simulink model "test_circuit_FMI"  (R2022a)
settings: Solver=FixedStepAuto  StartTime=0.0  StopTime=10.0  RelTol=1e-3
libraries: fl_lib x7, nesl_utility x5, spsControlledCurrentSourceLib x1, spsControlledVoltageSourceLib x1, spsCurrentMeasurementLib x1, spsGroundLib x1, spsParallelRLCBranchLib x1, spsSeriesRLCBranchLib x1, spsVoltageMeasurementLib x1, spspowerguiLib x1
(part 1 of 2)
settings Model: Creator=lordx  LastModifiedBy=lordx
settings SolverCC: ZeroCrossControl=EnableAll
settings OptimizationCC: DefaultParameterBehavior=Inlined  EnhancedBackFolding=on  PassReuseOutputArgsAs=Individual arguments  OptimizeBlockOrder=speed  DifferentSizesBufferReuse=on  OptimizationCustomize=off  EfficientTunableParamExpr=on
settings DebuggingCC: ParameterTunabilityLossMsg=error
settings HardwareCC: TargetBitPerPointer=64  TargetBitPerSizeT=64  TargetBitPerPtrDiffT=64  TargetLongLongMode=on  TargetIntDivRoundTo=Zero  TargetEndianess=LittleEndian  TargetWordSize=64  TargetHWDeviceType=MATLAB Host  ProdEqTarget=off
settings ModelReferenceCC: UpdateModelReferenceTargets=Force  EnableRefExpFcnMdlSchedulingChecks=off  ModelReferenceNumInstancesAllowed=Zero  PropagateSignalLabelsOutOfModel=off
settings SFSimCC: SimUserSources="\"F:\\GitHubRepos\\FMI_test_3\\test_circuit_FMI\\sources\\pm_printf.c\" \"F:\\GitHubRepos\\FMI_test_3\\test_circuit_FMI\\sources\\rt_backsubrr_dbl.c\" \"F:\\GitHubRepos\\FMI_test_3\\test_circuit_FMI\\sources\\rt_forwardsubrr_dbl.c\" \"F:\\GitHubRepos\\FMI_test_3\\test_circuit_FMI\\sources\\rt_lu_real.c\" \"F:\\GitHubRepos\\FMI_test_3\\test_circuit_FMI\\sources\\rt_matrixlib_dbl.c\" \"F:\\GitHubRepos\\FMI_test_3\\test_circuit_FMI\\sources\\test_circuit_FMI.c\" \"F:\\GitHubRepos\\FMI_test_3\\test_circuit_FMI\\sources\\test_circuit_FMI_data.c\" \"F:\\GitHubRepos\\FMI_test_3\\test_circuit_FMI\\sources\\RTWCG_FMU_util.c\" \"F:\\GitHubRepos\\FMI_test_3\\test_circuit_FMI\\sources\\test_circuit_FMI_fmu.c\" \"F:\\GitHubRepos\\FMI_test_3\\test_circuit_FMI\\sources\\ssc_sli_0267402d.c\" \"F:\\GitHubRepos\\FMI_test_3\\test_circuit_FMI\\sources\\ssc_sli_0763c151.c\" \"F:\\GitHubRepos\\FMI_test_3\\test_circuit_FMI\\sources\\ssc_sli_0bd269e6.c\" \"F:\\GitHubRepos\\FMI_test_3\\test_circuit_FMI\\sources\\ssc_sli_0d6d0780.c\" \"F:\\GitHubRepos\\FMI_test_3\\test_circuit_FMI\\sources\\ssc_sli_136b443c.c\" \"F:\\GitHubRepos\\FMI_test_3\\test_circuit_FMI\\sources\\ssc_sli_136f97a1.c\" \"F:\\GitHubRepos\\FMI_test_3\\test_circuit_FMI\\sources\\ssc_sli_140b3534.c\" \"F:\\GitHubRepos\\FMI_test_3\\test_circuit_FMI\\sources\\ssc_sli_15d5f6ce.c\" \"F:\\GitHubRepos\\FMI_test_3\\test_circuit_FMI\\sources\\ssc_sli_1c690f90.c\" \"F:\\GitHubRepos\\FMI_test_3\\test_circuit_FMI\\sources\\ssc_sli_1db813e8.c\" \"F:\\GitHubRepos\\FMI_test_3\\test_circuit_FMI\\sources\\ssc_sli_256cd4b6.c\" \"F:\\GitHubRepos\\FMI_test_3\\test_circuit_FMI\\sources\\ssc_sli_2bbd58a4.c\" \"F:\\GitHubRepos\\FMI_test_3\\test_circuit_FMI\\sources\\ssc_sli_2f6ea1cd.c\" \"F:\\GitHubRepos\\FMI_test_3\\test_circuit_FMI\\sources\\ssc_sli_360cfd63.c\" \"F:\\GitHubRepos\\FMI_test_3\\test_circuit_FMI\\sources\\ssc_sli_3fb4607e.c\" \"F:\\GitHubRepos\\FMI_test_3\\test_circuit_FMI\\sources\\ssc_sli_40d56d93.c\" \"F:\\GitHubRepos\\FMI_test_3\\test_circuit_FMI\\sources\\ssc_sli_42b14021.c\" \"F:\\GitHubRepos\\FMI_test_3\\test_circuit_FMI\\sources\\ssc_sli_43618287.c\" \"F:\\GitHubRepos\\FMI_test_3\\test_circuit_FMI\\sources\\ssc_sli_466b08dd.c\" \"F:\\GitHubRepos\\FMI_test_3\\test_circuit_FMI\\sources\\ssc_sli_496799bd.c\" \"F:\\GitHubRepos\\FMI_test_3\\test_circuit_FMI\\sources\\ssc_sli_4e028390.c\" \"F:\\GitHubRepos\\FMI_test_3\\test_circuit_FMI\\sources\\ssc_sli_51dbd3b5.c\" \"F:\\GitHubRepos\\FMI_test_3\\test_circuit_FMI\\sources\\ssc_sli_550a4805.c\" \"F:\\GitHubRepos\\FMI_test_3\\test_circuit_FMI\\sources\\ssc_sli_5a0cb974.c\" \"F:\\GitHubRepos\\FMI_test_3\\test_circuit_FMI\\sources\\ssc_sli_5d63aeeb.c\" \"F:\\GitHubRepos\\FMI_test_3\\test_circuit_FMI\\sources\\ssc_sli_62d81790.c\" \"F:\\GitHubRepos\\FMI_test_3\\test_circuit_FMI\\sources\\ssc_sli_77063d8b.c\" \"F:\\GitHubRepos\\FMI_test_3\\test_circuit_FMI\\sources\\ssc_sli_7a618260.c\" \"F:\\GitHubRepos\\FMI_test_3\\test_circuit_FMI\\sources\\ssc_sli_7f65db03.c\" \"F:\\GitHubRepos\\FMI_test_3\\test_circuit_FMI\\sources\\ssc_sli_880e593a.c\" \"F:\\GitHubRepos\\FMI_test_3\\test_circuit_FMI\\sources\\ssc_sli_89d0f30a.c\" \"F:\\GitHubRepos\\FMI_test_3\\test_circuit_FMI\\sources\\ssc_sli_8a64c4e2.c\" \"F:\\GitHubRepos\\FMI_test_3\\test_circuit_FMI\\sources\\ssc_sli_93019ea6.c\" \"F:\\GitHubRepos\\FMI_test_3\\test_circuit_FMI\\sources\\ssc_sli_9abcdb7f.c\" \"F:\\GitHubRepos\\FMI_test_3\\test_circuit_FMI\\sources\\ssc_sli_9b67747c.c\" \"F:\\GitHubRepos\\FMI_test_3\\test_circuit_FMI\\sources\\ssc_sli_9c030181.c\" \"F:\\GitHubRepos\\FMI_test_3\\test_circuit_FMI\\sources\\ssc_sli_c7dda239.c\" \"F:\\GitHubRepos\\FMI_test_3\\test_circuit_FMI\\sources\\ssc_sli_d064c978.c\" \"F:\\GitHubRepos\\FMI_test_3\\test_circuit_FMI\\sources\\ssc_sli_d80c44d2.c\" \"F:\\GitHubRepos\\FMI_test_3\\test_circuit_FMI\\sources\\ssc_sli_dcd66f69.c\" \"F:\\GitHubRepos\\FMI_test_3\\test_circuit_FMI\\sources\\ssc_sli_e66fe6d5.c\" \"F:\\GitHubRepos\\FMI_test_3\\test_circuit_FMI\\sources\\ssc_sli_e7b327bb.c\" \"F:\\GitHubRepos\\FMI_test_3\\test_circuit_FMI\\sources\\ssc_sli_eb0a5702.c\" \"F:\\GitHubRepos\\FMI_test_3\\test_circuit_FMI\\sources\\ssc_sli_edbee55c.c\" \"F:\\GitHubRepos\\FMI_test_3\\test_circuit_FMI\\sources\\ssc_sli_f6bd9cc8.c\" \"F:\\GitHubRepos\\FMI_test_3\\test_circuit_FMI\\sources\\ssc_sli_f9b5dbc5.c\" \"F:\\GitHubRepos\\FMI_test_3\\test_circuit_FMI\\sources\\ssc_sli_fa0ce53e.c\" \"F:\\GitHubRepos\\FMI_test_3\\test_circuit_FMI\\sources\\ssc_sli_fbdf29da.c\" \"F:\\GitHubRepos\\FMI_test_3\\test_circuit_FMI\\sources\\ssc_core_01dcc633.c\" \"F:\\GitHubRepos\\FMI_test_3\\test_circuit_FMI\\sources\\ssc_core_04da2c69.c\" \"F:\\GitHubRepos\\FMI_test_3\\test_circuit_FMI\\sources\\ssc_core_05058dd9.c\" \"F:\\GitHubRepos\\FMI_test_3\\test_circuit_FMI\\sources\\ssc_core_06ba68a6.c\" \"F:\\GitHubRepos\\FMI_test_3\\test_circuit_FMI\\sources\\ssc_core_09b5fa6e.c\" \"F:\\GitHubRepos\\FMI_test_3\\test_circuit_FMI\\sources\\ssc_core_0bd666aa.c\" \"F:\\GitHubRepos\\FMI_test_3\\test_circuit_FMI\\sources\\ssc_core_0d65be6c.c\" \"F:\\GitHubRepos\\FMI_test_3\\test_circuit_FMI\\sources\\ssc_core_0f019bd9.c\" \"F:\\GitHubRepos\\FMI_test_3\\test_circuit_FMI\\sources\\ssc_core_0f0420a6.c\" \"F:\\GitHubRepos\\FMI_test_3\\test_circuit_FMI\\sources\\ssc_core_18bf4d77.c\" \"F:\\GitHubRepos\\FMI_test_3\\test_circuit_FMI\\sources\\ssc_core_1b0cafd5.c\" \"F:\\GitHubRepos\\FMI_test_3\\test_circuit_FMI\\sources\\ssc_core_1c6b0332.c\" \"F:\\GitHubRepos\\FMI_test_3\\test_circuit_FMI\\sources\\ssc_core_1fd25120.c\" \"F:\\GitHubRepos\\FMI_test_3\\test_circuit_FMI\\sources\\ssc_core_24b4cdee.c\" \"F:\\GitHubRepos\\FMI_test_3\\test_circuit_FMI\\sources\\ssc_core_2568b075.c\" \"F:\\GitHubRepos\\FMI_test_3\\test_circuit_FMI\\sources\\ssc_core_280c0222.c\" \"F:\\GitHubRepos\\FMI_test_3\\test_circuit_FMI\\sources\\ssc_core_2cd54448.c\" \"F:\\GitHubRepos\\FMI_test_3\\test_circuit_FMI\\sources\\ssc_core_3169e4b7.c\" \"F:\\GitHubRepos\\FMI_test_3\\test_circuit_FMI\\sources\\ssc_core_32d8b307.c\" \"F:\\GitHubRepos\\FMI_test_3\\test_circuit_FMI\\sources\\ssc_core_3306c008.c\" \"F:\\GitHubRepos\\FMI_test_3\\test_circuit_FMI\\sources\\ssc_core_360a4baf.c\" \"F:\\GitHubRepos\\FMI_test_3\\test_circuit_FMI\\sources\\ssc_core_37d4ea84.c\" \"F:\\GitHubRepos\\FMI_test_3\\test_circuit_FMI\\sources\\ssc_core_40db642d.c\" \"F:\\GitHubRepos\\FMI_test_3\\test_circuit_FMI\\sources\\ssc_core_40dfdbdc.c\" \"F:\\GitHubRepos\\FMI_test_3\\test_circuit_FMI\\sources\\ssc_core_41017299.c\" \"F:\\GitHubRepos\\FMI_test_3\\test_circuit_FMI\\sources\\ssc_core_4666b45b.c\" \"F:\\GitHubRepos\\FMI_test_3\\test_circuit_FMI\\sources\\ssc_core_48b08af1.c\" \"F:\\GitHubRepos\\FMI_test_3\\test_circuit_FMI\\sources\\ssc_core_48b1386a.c\" \"F:\\GitHubRepos\\FMI_test_3\\test_circuit_FMI\\sources\\ssc_core_4965213d.c\" \"F:\\GitHubRepos\\FMI_test_3\\test_circuit_FMI\\sources\\ssc_core_4ad9135b.c\" \"F:\\GitHubRepos\\FMI_test_3\\test_circuit_FMI\\sources\\ssc_core_4db6bd68.c\" \"F:\\GitHubRepos\\FMI_test_3\\test_circuit_FMI\\sources\\ssc_core_4db86fcc.c\" \"F:\\GitHubRepos\\FMI_test_3\\test_circuit_FMI\\sources\\ssc_core_4e03e39d.c\" \"F:\\GitHubRepos\\FMI_test_3\\test_circuit_FMI\\sources\\ssc_core_4e04eecd.c\" \"F:\\GitHubRepos\\FMI_test_3\\test_circuit_FMI\\sources\\ssc_core_4e06e3bd.c\" \"F:\\GitHubRepos\\FMI_test_3\\test_circuit_FMI\\sources\\ssc_core_54d55ae9.c\" \"F:\\GitHubRepos\\FMI_test_3\\test_circuit_FMI\\sources\\ssc_core_5505224d.c\" \"F:\\GitHubRepos\\FMI_test_3\\test_circuit_FMI\\sources\\ssc_core_550b4c41.c\" \"F:\\GitHubRepos\\FMI_test_3\\test_circuit_FMI\\sources\\ssc_core_56b1a2bf.c\" \"F:\\GitHubRepos\\FMI_test_3\\test_circuit_FMI\\sources\\ssc_core_576cd129.c\" \"F:\\GitHubRepos\\FMI_test_3\\test_circuit_FMI\\sources\\ssc_core_59b034b8.c\" \"F:\\GitHubRepos\\FMI_test_3\\test_circuit_FMI\\sources\\ssc_core_5a046b27.c\" \"F:\\GitHubRepos\\FMI_test_3\\test_circuit_FMI\\sources\\ssc_core_5d6ba758.c\" \"F:\\GitHubRepos\\FMI_test_3\\test_circuit_FMI\\sources\\ssc_core_67d1f118.c\" \"F:\\GitHubRepos\\FMI_test_3\\test_circuit_FMI\\sources\\ssc_core_68da074b.c\" \"F:\\GitHubRepos\\FMI_test_3\\test_circuit_FMI\\sources\\ssc_core_6b663a17.c\" \"F:\\GitHubRepos\\FMI_test_3\\test_circuit_FMI\\sources\\ssc_core_6b6b89d2.c\" \"F:\\GitHubRepos\\FMI_test_3\\test_circuit_FMI\\sources\\ssc_core_6dd833f3.c\" \"F:\\GitHubRepos\\FMI_test_3\\test_circuit_FMI\\sources\\ssc_core_7209d3a5.c\" \"F:\\GitHubRepos\\FMI_test_3\\test_circuit_FMI\\sources\\ssc_core_73d9c2b7.c\" \"F:\\GitHubRepos\\FMI_test_3\\test_circuit_FMI\\sources\\ssc_core_76d825be.c\" \"F:\\GitHubRepos\\FMI_test_3\\test_circuit_FMI\\sources\\ssc_core_770cead7.c\" \"F:\\GitHubRepos\\FMI_test_3\\test_circuit_FMI\\sources\\ssc_core_79dd08ab.c\" \"F:\\GitHubRepos\\FMI_test_3\\test_circuit_FMI\\sources\\ssc_core_7a613edb.c\" \"F:\\GitHubRepos\\FMI_test_3\\test_circuit_FMI\\sources\\ssc_core_83db8762.c\" \"F:\\GitHubRepos\\FMI_test_3\\test_circuit_FMI\\sources\\ssc_core_856738f2.c\" \"F:\\GitHubRepos\\FMI_test_3\\test_circuit_FMI\\sources\\ssc_core_8569edc5.c\" \"F:\\GitHubRepos\\FMI_test_3\\test_circuit_FMI\\sources\\ssc_core_89d7fa79.c\" \"F:\\GitHubRepos\\FMI_test_3\\test_circuit_FMI\\sources\\ssc_core_8a6471dc.c\" \"F:\\GitHubRepos\\FMI_test_3\\test_circuit_FMI\\sources\\ssc_core_8cd9cb37.c\" \"F:\\GitHubRepos\\FMI_test_3\\test_circuit_FMI\\sources\\ssc_core_8d0064b8.c\" \"F:\\GitHubRepos\\FMI_test_3\\test_circuit_FMI\\sources\\ssc_core_96061071.c\" \"F:\\GitHubRepos\\FMI_test_3\\test_circuit_FMI\\sources\\ssc_core_97d767fe.c\" \"F:\\GitHubRepos\\FMI_test_3\\test_circuit_FMI\\sources\\ssc_core_990fe1a4.c\" \"F:\\GitHubRepos\\FMI_test_3\\test_circuit_FMI\\sources\\ssc_core_9b607b15.c\" \"F:\\GitHubRepos\\FMI_test_3\\test_circuit_FMI\\sources\\ssc_core_9b671e57.c\" \"F:\\GitHubRepos\\FMI_test_3\\test_circuit_FMI\\sources\\ssc_core_9c016445.c\" \"F:\\GitHubRepos\\FMI_test_3\\test_circuit_FMI\\sources\\ssc_core_9c01d168.c\" \"F:\\GitHubRepos\\FMI_test_3\\test_circuit_FMI\\sources\\ssc_core_9dd110ad.c\" \"F:\\GitHubRepos\\FMI_test_3\\test_circuit_FMI\\sources\\ssc_core_9fb0e229.c\" \"F:\\GitHubRepos\\FMI_test_3\\test_circuit_FMI\\sources\\ssc_core_9fb25b4f.c\" \"F:\\GitHubRepos\\FMI_test_3\\test_circuit_FMI\\sources\\ssc_core_9fb2e56c.c\" \"F:\\GitHubRepos\\FMI_test_3\\test_circuit_FMI\\sources\\ssc_core_a1d393be.c\" \"F:\\GitHubRepos\\FMI_test_3\\test_circuit_FMI\\sources\\ssc_core_a269ab09.c\" \"F:\\GitHubRepos\\FMI_test_3\\test_circuit_FMI\\sources\\ssc_core_a4d4c45e.c\" \"F:\\GitHubRepos\\FMI_test_3\\test_circuit_FMI\\sources\\ssc_core_a4da1d0a.c\" \"F:\\GitHubRepos\\FMI_test_3\\test_circuit_FMI\\sources\\ssc_core_a6b78ccc.c\" \"F:\\GitHubRepos\\FMI_test_3\\test_circuit_FMI\\sources\\ssc_core_a76299bc.c\" \"F:\\GitHubRepos\\FMI_test_3\\test_circuit_FMI\\sources\\ssc_core_a867d880.c\" \"F:\\GitHubRepos\\FMI_test_3\\test_circuit_FMI\\sources\\ssc_core_a9bbaecc.c\" \"F:\\GitHubRepos\\FMI_test_3\\test_circuit_FMI\\sources\\ssc_core_a9bf1ff2.c\" \"F:\\GitHubRepos\\FMI_test_3\\test_circuit_FMI\\sources\\ssc_core_aa09f23c.c\" \"F:\\GitHubRepos\\FMI_test_3\\test_circuit_FMI\\sources\\ssc_core_abd05c18.c\" \"F:\\GitHubRepos\\FMI_test_3\\test_circuit_FMI\\sources\\ssc_core_abd5e7b4.c\" \"F:\\GitHubRepos\\FMI_test_3\\test_circuit_FMI\\sources\\ssc_core_acb64294.c\" \"F:\\GitHubRepos\\FMI_test_3\\test_circuit_FMI\\sources\\ssc_core_acb6462e.c\" \"F:\\GitHubRepos\\FMI_test_3\\test_circuit_FMI\\sources\\ssc_core_b1038cbb.c\" \"F:\\GitHubRepos\\FMI_test_3\\test_circuit_FMI\\sources\\ssc_core_b10e34f4.c\" \"F:\\GitHubRepos\\FMI_test_3\\test_circuit_FMI\\sources\\ssc_core_b2b3b239.c\" \"F:\\GitHubRepos\\FMI_test_3\\test_circuit_FMI\\sources\\ssc_core_b369cd13.c\" \"F:\\GitHubRepos\\FMI_test_3\\test_circuit_FMI\\sources\\ssc_core_b402b40d.c\" \"F:\\GitHubRepos\\FMI_test_3\\test_circuit_FMI\\sources\\ssc_core_b7b88213.c\" \"F:\\GitHubRepos\\FMI_test_3\\test_circuit_FMI\\sources\\ssc_core_b96ebc21.c\" \"F:\\GitHubRepos\\FMI_test_3\\test_circuit_FMI\\sources\\ssc_core_bad68669.c\" \"F:\\GitHubRepos\\FMI_test_3\\test_circuit_FMI\\sources\\ssc_core_bc648043.c\" \"F:\\GitHubRepos\\FMI_test_3\\test_circuit_FMI\\sources\\ssc_core_bfdb08db.c\" \"F:\\GitHubRepos\\FMI_test_3\\test_circuit_FMI\\sources\\ssc_core_c3003040.c\" \"F:\\GitHubRepos\\FMI_test_3\\test_circuit_FMI\\sources\\ssc_core_c5b050d7.c\" \"F:\\GitHubRepos\\FMI_test_3\\test_circuit_FMI\\sources\\ssc_core_c5b63cb2.c\" \"F:\\GitHubRepos\\FMI_test_3\\test_circuit_FMI\\sources\\ssc_core_c607b660.c\" \"F:\\GitHubRepos\\FMI_test_3\\test_circuit_FMI\\sources\\ssc_core_c8d83e88.c\" \"F:\\GitHubRepos\\FMI_test_3\\test_circuit_FMI\\sources\\ssc_core_cab615c8.c\" \"F:\\GitHubRepos\\FMI_test_3\\test_circuit_FMI\\sources\\ssc_core_cabdc251.c\" \"F:\\GitHubRepos\\FMI_test_3\\test_circuit_FMI\\sources\\ssc_core_cc067f58.c\" \"F:\\GitHubRepos\\FMI_test_3\\test_circuit_FMI\\sources\\ssc_core_cc0bcab0.c\" \"F:\\GitHubRepos\\FMI_test_3\\test_circuit_FMI\\sources\\ssc_core_ce6a84bb.c\" \"F:\\GitHubRepos\\FMI_test_3\\test_circuit_FMI\\sources\\ssc_core_d06d763c.c\" \"F:\\GitHubRepos\\FMI_test_3\\test_circuit_FMI\\sources\\ssc_core_d3d34d7c.c\" \"F:\\GitHubRepos\\FMI_test_3\\test_circuit_FMI\\sources\\ssc_core_d4b9397b.c\" \"F:\\GitHubRepos\\FMI_test_3\\test_circuit_FMI\\sources\\ssc_core_d70a6a09.c\" \"F:\\GitHubRepos\\FMI_test_3\\test_circuit_FMI\\sources\\ssc_core_d807fa59.c\" \"F:\\GitHubRepos\\FMI_test_3\\test_circuit_FMI\\sources\\ssc_core_dcda6edd.c\" \"F:\\GitHubRepos\\FMI_test_3\\test_circuit_FMI\\sources\\ssc_core_deb7fd8d.c\" \"F:\\GitHubRepos\\FMI_test_3\\test_circuit_FMI\\sources\\ssc_core_e0d0866d.c\" \"F:\\GitHubRepos\\FMI_test_3\\test_circuit_FMI\\sources\\ssc_core_e2b61d72.c\" \"F:\\GitHubRepos\\FMI_test_3\\test_circuit_FMI\\sources\\ssc_core_e400c1c2.c\" \"F:\\GitHubRepos\\FMI_test_3\\test_circuit_FMI\\sources\\ssc_core_ead8f455.c\" \"F:\\GitHubRepos\\FMI_test_3\\test_circuit_FMI\\sources\\ssc_core_edb836de.c\" \"F:\\GitHubRepos\\FMI_test_3\\test_circuit_FMI\\sources\\ssc_core_ee000fbe.c\" \"F:\\GitHubRepos\\FMI_test_3\\test_circuit_FMI\\sources\\ssc_core_ee01086d.c\" \"F:\\GitHubRepos\\FMI_test_3\\test_circuit_FMI\\sources\\ssc_core_ee0f0141.c\" \"F:\\GitHubRepos\\FMI_test_3\\test_circuit_FMI\\sources\\ssc_core_f9b6dbed.c\" \"F:\\GitHubRepos\\FMI_test_3\\test_circuit_FMI\\sources\\ssc_core_fa09e9e6.c\" \"F:\\GitHubRepos\\FMI_test_3\\test_circuit_FMI\\sources\\ssc_core_fbd34e62.c\" \"F:\\GitHubRepos\\FMI_test_3\\test_circuit_FMI\\sources\\ssc_core_ff06d9a4.c\" \"F:\\GitHubRepos\\FMI_test_3\\test_circuit_FMI\\sources\\ssc_st_7cd93bb6.c\" \"F:\\GitHubRepos\\FMI_test_3\\test_circuit_FMI\\sources\\ssc_st_da6cd8f8.c\" \"F:\\GitHubRepos\\FMI_test_3\\test_circuit_FMI\\sources\\mc_026e4f4b.c\" \"F:\\GitHubRepos\\FMI_test_3\\test_circuit_FMI\\sources\\mc_03b98f6f.c\" \"F:\\GitHubRepos\\FMI_test_3\\test_circuit_FMI\\sources\\mc_0764157d.c\" \"F:\\GitHubRepos\\FMI_test_3\\test_circuit_FMI\\sources\\mc_0bd30dee.c\" \"F:\\GitHubRepos\\FMI_test_3\\test_circuit_FMI\\sources\\mc_0d6fd085.c\" \"F:\\GitHubRepos\\FMI_test_3\\test_circuit_FMI\\sources\\mc_0ed73c49.c\" \"F:\\GitHubRepos\\FMI_test_3\\test_circuit_FMI\\sources\\mc_0edc34e3.c\" \"F:\\GitHubRepos\\FMI_test_3\\test_circuit_FMI\\sources\\mc_10d4ab75.c\" \"F:\\GitHubRepos\\FMI_test_3\\test_circuit_FMI\\sources\\mc_11086079.c\" \"F:\\GitHubRepos\\FMI_test_3\\test_circuit_FMI\\sources\\mc_110e6c6c.c\" \"F:\\GitHubRepos\\FMI_test_3\\test_circuit_FMI\\sources\\mc_1407e917.c\" \"F:\\GitHubRepos\\FMI_test_3\\test_circuit_FMI\\sources\\mc_140e3c4c.c\" \"F:\\GitHubRepos\\FMI_test_3\\test_circuit_FMI\\sources\\mc_15d12d95.c\" \"F:\\GitHubRepos\\FMI_test_3\\test_circuit_FMI\\sources\\mc_15d828ca.c\" \"F:\\GitHubRepos\\FMI_test_3\\test_circuit_FMI\\sources\\mc_220ba961.c\" \"F:\\GitHubRepos\\FMI_test_3\\test_circuit_FMI\\sources\\mc_2565d6e0.c\" \"F:\\GitHubRepos\\FMI_test_3\\test_circuit_FMI\\sources\\mc_2a642f54.c\" \"F:\\GitHubRepos\\FMI_test_3\\test_circuit_FMI\\sources\\mc_2a6a9b24.c\" \"F:\\GitHubRepos\\FMI_test_3\\test_circuit_FMI\\sources\\mc_2a6b417d.c\" \"F:\\GitHubRepos\\FMI_test_3\\test_circuit_FMI\\sources\\mc_2bbf87e3.c\" \"F:\\GitHubRepos\\FMI_test_3\\test_circuit_FMI\\sources\\mc_2cdc96b4.c\" \"F:\\GitHubRepos\\FMI_test_3\\test_circuit_FMI\\sources\\mc_32d501e3.c\" \"F:\\GitHubRepos\\FMI_test_3\\test_circuit_FMI\\sources\\mc_32dc008a.c\" \"F:\\GitHubRepos\\FMI_test_3\\test_circuit_FMI\\sources\\mc_3b6a945d.c\" \"F:\\GitHubRepos\\FMI_test_3\\test_circuit_FMI\\sources\\mc_3e66abdf.c\" \"F:\\GitHubRepos\\FMI_test_3\\test_circuit_FMI\\sources\\mc_4105189f.c\" \"F:\\GitHubRepos\\FMI_test_3\\test_circuit_FMI\\sources\\mc_47b8cebe.c\" \"F:\\GitHubRepos\\FMI_test_3\\test_circuit_FMI\\sources\\mc_47b91db1.c\" \"F:\\GitHubRepos\\FMI_test_3\\test_circuit_FMI\\sources\\mc_4b0301c6.c\" \"F:\\GitHubRepos\\FMI_test_3\\test_circuit_FMI\\sources\\mc_4c6117e3.c\" \"F:\\GitHubRepos\\FMI_test_3\\test_circuit_FMI\\sources\\mc_51d4094e.c\" \"F:\\GitHubRepos\\FMI_test_3\\test_circuit_FMI\\sources\\mc_52623861.c\" \"F:\\GitHubRepos\\FMI_test_3\\test_circuit_FMI\\sources\\mc_52688a58.c\" \"F:\\GitHubRepos\\FMI_test_3\\test_circuit_FMI\\sources\\mc_53b1fc84.c\" \"F:\\GitHubRepos\\FMI_test_3\\test_circuit_FMI\\sources\\mc_53b6fcf3.c\" \"F:\\GitHubRepos\\FMI_test_3\\test_circuit_FMI\\sources\\mc_550847c3.c\" \"F:\\GitHubRepos\\FMI_test_3\\test_circuit_FMI\\sources\\mc_5766048f.c\" \"F:\\GitHubRepos\\FMI_test_3\\test_circuit_FMI\\sources\\mc_59b6e413.c\" \"F:\\GitHubRepos\\FMI_test_3\\test_circuit_FMI\\sources\\mc_5bd2c9c1.c\" \"F:\\GitHubRepos\\FMI_test_3\\test_circuit_FMI\\sources\\mc_5d65cd86.c\" \"F:\\GitHubRepos\\FMI_test_3\\test_circuit_FMI\\sources\\mc_5edd42ef.c\" \"F:\\GitHubRepos\\FMI_test_3\\test_circuit_FMI\\sources\\mc_630208f8.c\" \"F:\\GitHubRepos\\FMI_test_3\\test_circuit_FMI\\sources\\mc_630dda0e.c\" \"F:\\GitHubRepos\\FMI_test_3\\test_circuit_FMI\\sources\\mc_67da200d.c\" \"F:\\GitHubRepos\\FMI_test_3\\test_circuit_FMI\\sources\\mc_67da4f41.c\" \"F:\\GitHubRepos\\FMI_test_3\\test_circuit_FMI\\sources\\mc_6b6d311a.c\" \"F:\\GitHubRepos\\FMI_test_3\\test_circuit_FMI\\sources\\mc_6e61d16c.c\" \"F:\\GitHubRepos\\FMI_test_3\\test_circuit_FMI\\sources\\mc_6fb1c336.c\" \"F:\\GitHubRepos\\FMI_test_3\\test_circuit_FMI\\sources\\mc_7207b6f4.c\" \"F:\\GitHubRepos\\FMI_test_3\\test_circuit_FMI\\sources\\mc_7809a65c.c\" \"F:\\GitHubRepos\\FMI_test_3\\test_circuit_FMI\\sources\\mc_7a613aec.c\" \"F:\\GitHubRepos\\FMI_test_3\\test_circuit_FMI\\sources\\mc_7bbf41f0.c\" \"F:\\GitHubRepos\\FMI_test_3\\test_circuit_FMI\\sources\\mc_7cd58f0b.c\" \"F:\\GitHubRepos\\FMI_test_3\\test_circuit_FMI\\sources\\mc_7cdbe436.c\" \"F:\\GitHubRepos\\FMI_test_3\\test_circuit_FMI\\sources\\mc_7d0547c8.c\" \"F:\\GitHubRepos\\FMI_test_3\\test_circuit_FMI\\sources\\mc_7d099de7.c\" \"F:\\GitHubRepos\\FMI_test_3\\test_circuit_FMI\\sources\\mc_7eb21b39.c\" \"F:\\GitHubRepos\\FMI_test_3\\test_circuit_FMI\\sources\\mc_81b0ada5.c\" \"F:\\GitHubRepos\\FMI_test_3\\test_circuit_FMI\\sources\\mc_81b5717e.c\" \"F:\\GitHubRepos\\FMI_test_3\\test_circuit_FMI\\sources\\mc_81bc7943.c\" \"F:\\GitHubRepos\\FMI_test_3\\test_circuit_FMI\\sources\\mc_870ec75e.c\" \"F:\\GitHubRepos\\FMI_test_3\\test_circuit_FMI\\sources\\mc_89d597cf.c\" \"F:\\GitHubRepos\\FMI_test_3\\test_circuit_FMI\\sources\\mc_90b6aa0a.c\" \"F:\\GitHubRepos\\FMI_test_3\\test_circuit_FMI\\sources\\mc_95b62b73.c\" \"F:\\GitHubRepos\\FMI_test_3\\test_circuit_FMI\\sources\\mc_9ab7d9b0.c\" \"F:\\GitHubRepos\\FMI_test_3\\test_circuit_FMI\\sources\\mc_9b6376d1.c\" \"F:\\GitHubRepos\\FMI_test_3\\test_circuit_FMI\\sources\\mc_9b6c1529.c\" \"F:\\GitHubRepos\\FMI_test_3\\test_circuit_FMI\\sources\\mc_a2647600.c\" \"F:\\GitHubRepos\\FMI_test_3\\test_circuit_FMI\\sources\\mc_a26bab1a.c\" \"F:\\GitHubRepos\\FMI_test_3\\test_circuit_FMI\\sources\\mc_a3b90582.c\" \"F:\\GitHubRepos\\FMI_test_3\\test_circuit_FMI\\sources\\mc_a6b5ed24.c\" \"F:\\GitHubRepos\\FMI_test_3\\test_circuit_FMI\\sources\\mc_a7684938.c\" \"F:\\GitHubRepos\\FMI_test_3\\test_circuit_FMI\\sources\\mc_a865d1dd.c\" \"F:\\GitHubRepos\\FMI_test_3\\test_circuit_FMI\\sources\\mc_acb3fad7.c\" \"F:\\GitHubRepos\\FMI_test_3\\test_circuit_FMI\\sources\\mc_af0bc203.c\" \"F:\\GitHubRepos\\FMI_test_3\\test_circuit_FMI\\sources\\mc_af0cc4c9.c\" \"F:\\GitHubRepos\\FMI_test_3\\test_circuit_FMI\\sources\\mc_b0de9cbc.c\" \"F:\\GitHubRepos\\FMI_test_3\\test_circuit_FMI\\sources\\mc_b2b86ae3.c\" \"F:\\GitHubRepos\\FMI_test_3\\test_circuit_FMI\\sources\\mc_b362c5eb.c\" \"F:\\GitHubRepos\\FMI_test_3\\test_circuit_FMI\\sources\\mc_b7b03d44.c\" \"F:\\GitHubRepos\\FMI_test_3\\test_circuit_FMI\\sources\\mc_b96a0bad.c\" \"F:\\GitHubRepos\\FMI_test_3\\test_circuit_FMI\\sources\\mc_bb0520ee.c\" \"F:\\GitHubRepos\\FMI_test_3\\test_circuit_FMI\\sources\\mc_bdbb9b78.c\" \"F:\\GitHubRepos\\FMI_test_3\\test_circuit_FMI\\sources\\mc_c2dbf4b2.c\" \"F:\\GitHubRepos\\FMI_test_3\\test_circuit_FMI\\sources\\mc_c8d25d23.c\" \"F:\\GitHubRepos\\FMI_test_3\\test_circuit_FMI\\sources\\mc_cab8a1f9.c\" \"F:\\GitHubRepos\\FMI_test_3\\test_circuit_FMI\\sources\\mc_ce6656ce.c\" \"F:\\GitHubRepos\\FMI_test_3\\test_circuit_FMI\\sources\\mc_d20085b7.c\" \"F:\\GitHubRepos\\FMI_test_3\\test_circuit_FMI\\sources\\mc_d9d38185.c\" \"F:\\GitHubRepos\\FMI_test_3\\test_circuit_FMI\\sources\\mc_dbbb14d2.c\" \"F:\\GitHubRepos\\FMI_test_3\\test_circuit_FMI\\sources\\mc_dcdddfae.c\" \"F:\\GitHubRepos\\FMI_test_3\\test_circuit_FMI\\sources\\mc_debb448f.c\" \"F:\\GitHubRepos\\FMI_test_3\\test_circuit_FMI\\sources\\mc_e7b99cf6.c\" \"F:\\GitHubRepos\\FMI_test_3\\test_circuit_FMI\\sources\\mc_e7bc2f1a.c\" \"F:\\GitHubRepos\\FMI_test_3\\test_circuit_FMI\\sources\\mc_e9661c4a.c\" \"F:\\GitHubRepos\\FMI_test_3\\test_circuit_FMI\\sources\\mc_e969ae87.c\" \"F:\\GitHubRepos\\FMI_test_3\\test_circuit_FMI\\sources\\mc_edbf543c.c\" \"F:\\GitHubRepos\\FMI_test_3\\test_circuit_FMI\\sources\\mc_ee000fbe.c\" \"F:\\GitHubRepos\\FMI_test_3\\test_circuit_FMI\\sources\\mc_efdea3a7.c\" \"F:\\GitHubRepos\\FMI_test_3\\test_circuit_FMI\\sources\\mc_f0012953.c\" \"F:\\GitHubRepos\\FMI_test_3\\test_circuit_FMI\\sources\\mc_f00d2f9b.c\" \"F:\\GitHubRepos\\FMI_test_3\\test_circuit_FMI\\sources\\mc_f3be157c.c\" \"F:\\GitHubRepos\\FMI_test_3\\test_circuit_FMI\\sources\\mc_fbd54145.c\" \"F:\\GitHubRepos\\FMI_test_3\\test_circuit_FMI\\sources\\mc_fcb15a9b.c\" \"F:\\GitHubRepos\\FMI_test_3\\test_circuit_FMI\\sources\\mc_fd619d14.c\" \"F:\\GitHubRepos\\FMI_test_3\\test_circuit_FMI\\sources\\mc_fd6341bb.c\" \"F:\\GitHubRepos\\FMI_test_3\\test_circuit_FMI\\sources\\ex_04d5441d.c\" \"F:\\GitHubRepos\\FMI_test_3\\test_circuit_FMI\\sources\\ex_0d6d0784.c\" \"F:\\GitHubRepos\\FMI_test_3\\test_circuit_FMI\\sources\\ex_136645f8.c\" \"F:\\GitHubRepos\\FMI_test_3\\test_circuit_FMI\\sources\\ex_17bc61ac.c\" \"F:\\GitHubRepos\\FMI_test_3\\test_circuit_FMI\\sources\\ex_18b4440a.c\" \"F:\\GitHubRepos\\FMI_test_3\\test_circuit_FMI\\sources\\ex_1b03ca17.c\" \"F:\\GitHubRepos\\FMI_test_3\\test_circuit_FMI\\sources\\ex_2ebcd5b2.c\" \"F:\\GitHubRepos\\FMI_test_3\\test_circuit_FMI\\sources\\ex_316a81de.c\" \"F:\\GitHubRepos\\FMI_test_3\\test_circuit_FMI\\sources\\ex_36012fa7.c\" \"F:\\GitHubRepos\\FMI_test_3\\test_circuit_FMI\\sources\\ex_40d5be33.c\" \"F:\\GitHubRepos\\FMI_test_3\\test_circuit_FMI\\sources\\ex_47b11894.c\" \"F:\\GitHubRepos\\FMI_test_3\\test_circuit_FMI\\sources\\ex_57660158.c\" \"F:\\GitHubRepos\\FMI_test_3\\test_circuit_FMI\\sources\\ex_690b7cd0.c\" \"F:\\GitHubRepos\\FMI_test_3\\test_circuit_FMI\\sources\\ex_6dd8e72d.c\" \"F:\\GitHubRepos\\FMI_test_3\\test_circuit_FMI\\sources\\ex_770385e6.c\" \"F:\\GitHubRepos\\FMI_test_3\\test_circuit_FMI\\sources\\ex_79d100f1.c\" \"F:\\GitHubRepos\\FMI_test_3\\test_circuit_FMI\\sources\\ex_8a6fc761.c\" \"F:\\GitHubRepos\\FMI_test_3\\test_circuit_FMI\\sources\\ex_98d223a6.c\" \"F:\\GitHubRepos\\FMI_test_3\\test_circuit_FMI\\sources\\ex_aed5de1e.c\" \"F:\\GitHubRepos\\FMI_test_3\\test_circuit_FMI\\sources\\ex_b2b40ad5.c\" \"F:\\GitHubRepos\\FMI_test_3\\test_circuit_FMI\\sources\\ex_bb0efd4b.c\" \"F:\\GitHubRepos\\FMI_test_3\\test_circuit_FMI\\sources\\ex_bfdb009c.c\" \"F:\\GitHubRepos\\FMI_test_3\\test_circuit_FMI\\sources\\ex_c9069dae.c\" \"F:\\GitHubRepos\\FMI_test_3\\test_circuit_FMI\\sources\\ex_d9d686a8.c\" \"F:\\GitHubRepos\\FMI_test_3\\test_circuit_FMI\\sources\\ex_debffef2.c\" \"F:\\GitHubRepos\\FMI_test_3\\test_circuit_FMI\\sources\\ex_e40d74b8.c\" \"F:\\GitHubRepos\\FMI_test_3\\test_circuit_FMI\\sources\\ex_eb0d559b.c\" \"F:\\GitHubRepos\\FMI_test_3\\test_circuit_FMI\\sources\\ex_f6bb4c2d.c\" \"F:\\GitHubRepos\\FMI_test_3\\test_circuit_FMI\\sources\\ex_f866102d.c\" \"F:\\GitHubRepos\\FMI_test_3\\test_circuit_FMI\\sources\\slu_stubbed_definitions.c\" \"F:\\GitHubRepos\\FMI_test_3\\test_circuit_FMI\\sources\\pm_09bc42e2.c\" \"F:\\GitHubRepos\\FMI_test_3\\test_circuit_FMI\\sources\\pm_14098e54.c\" \"F:\\GitHubRepos\\FMI_test_3\\test_circuit_FMI\\sources\\pm_26dc3230.c\" \"F:\\GitHubRepos\\FMI_test_3\\test_circuit_FMI\\sources\\pm_4fd5f5b9.c\" \"F:\\GitHubRepos\\FMI_test_3\\test_circuit_FMI\\sources\\pm_fed8c2c9.c\""  SimUserIncludeDirs="\"D:\\Program Files\\Matlab\\rtw\\c\\FMIKit-Simulink-3.0\" \"D:\\Program Files\\Matlab\\rtw\\c\\FMIKit-Simulink-3.0\\include\" \"F:\\GitHubRepos\\FMI_test_3\\test_circuit_FMI\\sources\""  MATLABDynamicMemAlloc=off
settings RTWCC: SystemTargetFile=ert.tlc  TemplateMakefile=ert_default_tmf  GenerateReport=on  RetainRTWFile=on  CustomInclude="\"D:\\Program Files\\Matlab\\rtw\\c\\FMIKit-Simulink-3.0\" \"D:\\Program Files\\Matlab\\rtw\\c\\FMIKit-Simulink-3.0\\include\" \"F:\\GitHubRepos\\FMI_test_3\\test_circuit_FMI\\sources\""  CustomSource="\"F:\\GitHubRepos\\FMI_test_3\\test_circuit_FMI\\sources\\pm_printf.c\" \"F:\\GitHubRepos\\FMI_test_3\\test_circuit_FMI\\sources\\rt_backsubrr_dbl.c\" \"F:\\GitHubRepos\\FMI_test_3\\test_circuit_FMI\\sources\\rt_forwardsubrr_dbl.c\" \"F:\\GitHubRepos\\FMI_test_3\\test_circuit_FMI\\sources\\rt_lu_real.c\" \"F:\\GitHubRepos\\FMI_test_3\\test_circuit_FMI\\sources\\rt_matrixlib_dbl.c\" \"F:\\GitHubRepos\\FMI_test_3\\test_circuit_FMI\\sources\\test_circuit_FMI.c\" \"F:\\GitHubRepos\\FMI_test_3\\test_circuit_FMI\\sources\\test_circuit_FMI_data.c\" \"F:\\GitHubRepos\\FMI_test_3\\test_circuit_FMI\\sources\\RTWCG_FMU_util.c\" \"F:\\GitHubRepos\\FMI_test_3\\test_circuit_FMI\\sources\\test_circuit_FMI_fmu.c\" \"F:\\GitHubRepos\\FMI_test_3\\test_circuit_FMI\\sources\\ssc_sli_0267402d.c\" \"F:\\GitHubRepos\\FMI_test_3\\test_circuit_FMI\\sources\\ssc_sli_0763c151.c\" \"F:\\GitHubRepos\\FMI_test_3\\test_circuit_FMI\\sources\\ssc_sli_0bd269e6.c\" \"F:\\GitHubRepos\\FMI_test_3\\test_circuit_FMI\\sources\\ssc_sli_0d6d0780.c\" \"F:\\GitHubRepos\\FMI_test_3\\test_circuit_FMI\\sources\\ssc_sli_136b443c.c\" \"F:\\GitHubRepos\\FMI_test_3\\test_circuit_FMI\\sources\\ssc_sli_136f97a1.c\" \"F:\\GitHubRepos\\FMI_test_3\\test_circuit_FMI\\sources\\ssc_sli_140b3534.c\" \"F:\\GitHubRepos\\FMI_test_3\\test_circuit_FMI\\sources\\ssc_sli_15d5f6ce.c\" \"F:\\GitHubRepos\\FMI_test_3\\test_circuit_FMI\\sources\\ssc_sli_1c690f90.c\" \"F:\\GitHubRepos\\FMI_test_3\\test_circuit_FMI\\sources\\ssc_sli_1db813e8.c\" \"F:\\GitHubRepos\\FMI_test_3\\test_circuit_FMI\\sources\\ssc_sli_256cd4b6.c\" \"F:\\GitHubRepos\\FMI_test_3\\test_circuit_FMI\\sources\\ssc_sli_2bbd58a4.c\" \"F:\\GitHubRepos\\FMI_test_3\\test_circuit_FMI\\sources\\ssc_sli_2f6ea1cd.c\" \"F:\\GitHubRepos\\FMI_test_3\\test_circuit_FMI\\sources\\ssc_sli_360cfd63.c\" \"F:\\GitHubRepos\\FMI_test_3\\test_circuit_FMI\\sources\\ssc_sli_3fb4607e.c\" \"F:\\GitHubRepos\\FMI_test_3\\test_circuit_FMI\\sources\\ssc_sli_40d56d93.c\" \"F:\\GitHubRepos\\FMI_test_3\\test_circuit_FMI\\sources\\ssc_sli_42b14021.c\" \"F:\\GitHubRepos\\FMI_test_3\\test_circuit_FMI\\sources\\ssc_sli_43618287.c\" \"F:\\GitHubRepos\\FMI_test_3\\test_circuit_FMI\\sources\\ssc_sli_466b08dd.c\" \"F:\\GitHubRepos\\FMI_test_3\\test_circuit_FMI\\sources\\ssc_sli_496799bd.c\" \"F:\\GitHubRepos\\FMI_test_3\\test_circuit_FMI\\sources\\ssc_sli_4e028390.c\" \"F:\\GitHubRepos\\FMI_test_3\\test_circuit_FMI\\sources\\ssc_sli_51dbd3b5.c\" \"F:\\GitHubRepos\\FMI_test_3\\test_circuit_FMI\\sources\\ssc_sli_550a4805.c\" \"F:\\GitHubRepos\\FMI_test_3\\test_circuit_FMI\\sources\\ssc_sli_5a0cb974.c\" \"F:\\GitHubRepos\\FMI_test_3\\test_circuit_FMI\\sources\\ssc_sli_5d63aeeb.c\" \"F:\\GitHubRepos\\FMI_test_3\\test_circuit_FMI\\sources\\ssc_sli_62d81790.c\" \"F:\\GitHubRepos\\FMI_test_3\\test_circuit_FMI\\sources\\ssc_sli_77063d8b.c\" \"F:\\GitHubRepos\\FMI_test_3\\test_circuit_FMI\\sources\\ssc_sli_7a618260.c\" \"F:\\GitHubRepos\\FMI_test_3\\test_circuit_FMI\\sources\\ssc_sli_7f65db03.c\" \"F:\\GitHubRepos\\FMI_test_3\\test_circuit_FMI\\sources\\ssc_sli_880e593a.c\" \"F:\\GitHubRepos\\FMI_test_3\\test_circuit_FMI\\sources\\ssc_sli_89d0f30a.c\" \"F:\\GitHubRepos\\FMI_test_3\\test_circuit_FMI\\sources\\ssc_sli_8a64c4e2.c\" \"F:\\GitHubRepos\\FMI_test_3\\test_circuit_FMI\\sources\\ssc_sli_93019ea6.c\" \"F:\\GitHubRepos\\FMI_test_3\\test_circuit_FMI\\sources\\ssc_sli_9abcdb7f.c\" \"F:\\GitHubRepos\\FMI_test_3\\test_circuit_FMI\\sources\\ssc_sli_9b67747c.c\" \"F:\\GitHubRepos\\FMI_test_3\\test_circuit_FMI\\sources\\ssc_sli_9c030181.c\" \"F:\\GitHubRepos\\FMI_test_3\\test_circuit_FMI\\sources\\ssc_sli_c7dda239.c\" \"F:\\GitHubRepos\\FMI_test_3\\test_circuit_FMI\\sources\\ssc_sli_d064c978.c\" \"F:\\GitHubRepos\\FMI_test_3\\test_circuit_FMI\\sources\\ssc_sli_d80c44d2.c\" \"F:\\GitHubRepos\\FMI_test_3\\test_circuit_FMI\\sources\\ssc_sli_dcd66f69.c\" \"F:\\GitHubRepos\\FMI_test_3\\test_circuit_FMI\\sources\\ssc_sli_e66fe6d5.c\" \"F:\\GitHubRepos\\FMI_test_3\\test_circuit_FMI\\sources\\ssc_sli_e7b327bb.c\" \"F:\\GitHubRepos\\FMI_test_3\\test_circuit_FMI\\sources\\ssc_sli_eb0a5702.c\" \"F:\\GitHubRepos\\FMI_test_3\\test_circuit_FMI\\sources\\ssc_sli_edbee55c.c\" \"F:\\GitHubRepos\\FMI_test_3\\test_circuit_FMI\\sources\\ssc_sli_f6bd9cc8.c\" \"F:\\GitHubRepos\\FMI_test_3\\test_circuit_FMI\\sources\\ssc_sli_f9b5dbc5.c\" \"F:\\GitHubRepos\\FMI_test_3\\test_circuit_FMI\\sources\\ssc_sli_fa0ce53e.c\" \"F:\\GitHubRepos\\FMI_test_3\\test_circuit_FMI\\sources\\ssc_sli_fbdf29da.c\" \"F:\\GitHubRepos\\FMI_test_3\\test_circuit_FMI\\sources\\ssc_core_01dcc633.c\" \"F:\\GitHubRepos\\FMI_test_3\\test_circuit_FMI\\sources\\ssc_core_04da2c69.c\" \"F:\\GitHubRepos\\FMI_test_3\\test_circuit_FMI\\sources\\ssc_core_05058dd9.c\" \"F:\\GitHubRepos\\FMI_test_3\\test_circuit_FMI\\sources\\ssc_core_06ba68a6.c\" \"F:\\GitHubRepos\\FMI_test_3\\test_circuit_FMI\\sources\\ssc_core_09b5fa6e.c\" \"F:\\GitHubRepos\\FMI_test_3\\test_circuit_FMI\\sources\\ssc_core_0bd666aa.c\" \"F:\\GitHubRepos\\FMI_test_3\\test_circuit_FMI\\sources\\ssc_core_0d65be6c.c\" \"F:\\GitHubRepos\\FMI_test_3\\test_circuit_FMI\\sources\\ssc_core_0f019bd9.c\" \"F:\\GitHubRepos\\FMI_test_3\\test_circuit_FMI\\sources\\ssc_core_0f0420a6.c\" \"F:\\GitHubRepos\\FMI_test_3\\test_circuit_FMI\\sources\\ssc_core_18bf4d77.c\" \"F:\\GitHubRepos\\FMI_test_3\\test_circuit_FMI\\sources\\ssc_core_1b0cafd5.c\" \"F:\\GitHubRepos\\FMI_test_3\\test_circuit_FMI\\sources\\ssc_core_1c6b0332.c\" \"F:\\GitHubRepos\\FMI_test_3\\test_circuit_FMI\\sources\\ssc_core_1fd25120.c\" \"F:\\GitHubRepos\\FMI_test_3\\test_circuit_FMI\\sources\\ssc_core_24b4cdee.c\" \"F:\\GitHubRepos\\FMI_test_3\\test_circuit_FMI\\sources\\ssc_core_2568b075.c\" \"F:\\GitHubRepos\\FMI_test_3\\test_circuit_FMI\\sources\\ssc_core_280c0222.c\" \"F:\\GitHubRepos\\FMI_test_3\\test_circuit_FMI\\sources\\ssc_core_2cd54448.c\" \"F:\\GitHubRepos\\FMI_test_3\\test_circuit_FMI\\sources\\ssc_core_3169e4b7.c\" \"F:\\GitHubRepos\\FMI_test_3\\test_circuit_FMI\\sources\\ssc_core_32d8b307.c\" \"F:\\GitHubRepos\\FMI_test_3\\test_circuit_FMI\\sources\\ssc_core_3306c008.c\" \"F:\\GitHubRepos\\FMI_test_3\\test_circuit_FMI\\sources\\ssc_core_360a4baf.c\" \"F:\\GitHubRepos\\FMI_test_3\\test_circuit_FMI\\sources\\ssc_core_37d4ea84.c\" \"F:\\GitHubRepos\\FMI_test_3\\test_circuit_FMI\\sources\\ssc_core_40db642d.c\" \"F:\\GitHubRepos\\FMI_test_3\\test_circuit_FMI\\sources\\ssc_core_40dfdbdc.c\" \"F:\\GitHubRepos\\FMI_test_3\\test_circuit_FMI\\sources\\ssc_core_41017299.c\" \"F:\\GitHubRepos\\FMI_test_3\\test_circuit_FMI\\sources\\ssc_core_4666b45b.c\" \"F:\\GitHubRepos\\FMI_test_3\\test_circuit_FMI\\sources\\ssc_core_48b08af1.c\" \"F:\\GitHubRepos\\FMI_test_3\\test_circuit_FMI\\sources\\ssc_core_48b1386a.c\" \"F:\\GitHubRepos\\FMI_test_3\\test_circuit_FMI\\sources\\ssc_core_4965213d.c\" \"F:\\GitHubRepos\\FMI_test_3\\test_circuit_FMI\\sources\\ssc_core_4ad9135b.c\" \"F:\\GitHubRepos\\FMI_test_3\\test_circuit_FMI\\sources\\ssc_core_4db6bd68.c\" \"F:\\GitHubRepos\\FMI_test_3\\test_circuit_FMI\\sources\\ssc_core_4db86fcc.c\" \"F:\\GitHubRepos\\FMI_test_3\\test_circuit_FMI\\sources\\ssc_core_4e03e39d.c\" \"F:\\GitHubRepos\\FMI_test_3\\test_circuit_FMI\\sources\\ssc_core_4e04eecd.c\" \"F:\\GitHubRepos\\FMI_test_3\\test_circuit_FMI\\sources\\ssc_core_4e06e3bd.c\" \"F:\\GitHubRepos\\FMI_test_3\\test_circuit_FMI\\sources\\ssc_core_54d55ae9.c\" \"F:\\GitHubRepos\\FMI_test_3\\test_circuit_FMI\\sources\\ssc_core_5505224d.c\" \"F:\\GitHubRepos\\FMI_test_3\\test_circuit_FMI\\sources\\ssc_core_550b4c41.c\" \"F:\\GitHubRepos\\FMI_test_3\\test_circuit_FMI\\sources\\ssc_core_56b1a2bf.c\" \"F:\\GitHubRepos\\FMI_test_3\\test_circuit_FMI\\sources\\ssc_core_576cd129.c\" \"F:\\GitHubRepos\\FMI_test_3\\test_circuit_FMI\\sources\\ssc_core_59b034b8.c\" \"F:\\GitHubRepos\\FMI_test_3\\test_circuit_FMI\\sources\\ssc_core_5a046b27.c\" \"F:\\GitHubRepos\\FMI_test_3\\test_circuit_FMI\\sources\\ssc_core_5d6ba758.c\" \"F:\\GitHubRepos\\FMI_test_3\\test_circuit_FMI\\sources\\ssc_core_67d1f118.c\" \"F:\\GitHubRepos\\FMI_test_3\\test_circuit_FMI\\sources\\ssc_core_68da074b.c\" \"F:\\GitHubRepos\\FMI_test_3\\test_circuit_FMI\\sources\\ssc_core_6b663a17.c\" \"F:\\GitHubRepos\\FMI_test_3\\test_circuit_FMI\\sources\\ssc_core_6b6b89d2.c\" \"F:\\GitHubRepos\\FMI_test_3\\test_circuit_FMI\\sources\\ssc_core_6dd833f3.c\" \"F:\\GitHubRepos\\FMI_test_3\\test_circuit_FMI\\sources\\ssc_core_7209d3a5.c\" \"F:\\GitHubRepos\\FMI_test_3\\test_circuit_FMI\\sources\\ssc_core_73d9c2b7.c\" \"F:\\GitHubRepos\\FMI_test_3\\test_circuit_FMI\\sources\\ssc_core_76d825be.c\" \"F:\\GitHubRepos\\FMI_test_3\\test_circuit_FMI\\sources\\ssc_core_770cead7.c\" \"F:\\GitHubRepos\\FMI_test_3\\test_circuit_FMI\\sources\\ssc_core_79dd08ab.c\" \"F:\\GitHubRepos\\FMI_test_3\\test_circuit_FMI\\sources\\ssc_core_7a613edb.c\" \"F:\\GitHubRepos\\FMI_test_3\\test_circuit_FMI\\sources\\ssc_core_83db8762.c\" \"F:\\GitHubRepos\\FMI_test_3\\test_circuit_FMI\\sources\\ssc_core_856738f2.c\" \"F:\\GitHubRepos\\FMI_test_3\\test_circuit_FMI\\sources\\ssc_core_8569edc5.c\" \"F:\\GitHubRepos\\FMI_test_3\\test_circuit_FMI\\sources\\ssc_core_89d7fa79.c\" \"F:\\GitHubRepos\\FMI_test_3\\test_circuit_FMI\\sources\\ssc_core_8a6471dc.c\" \"F:\\GitHubRepos\\FMI_test_3\\test_circuit_FMI\\sources\\ssc_core_8cd9cb37.c\" \"F:\\GitHubRepos\\FMI_test_3\\test_circuit_FMI\\sources\\ssc_core_8d0064b8.c\" \"F:\\GitHubRepos\\FMI_test_3\\test_circuit_FMI\\sources\\ssc_core_96061071.c\" \"F:\\GitHubRepos\\FMI_test_3\\test_circuit_FMI\\sources\\ssc_core_97d767fe.c\" \"F:\\GitHubRepos\\FMI_test_3\\test_circuit_FMI\\sources\\ssc_core_990fe1a4.c\" \"F:\\GitHubRepos\\FMI_test_3\\test_circuit_FMI\\sources\\ssc_core_9b607b15.c\" \"F:\\GitHubRepos\\FMI_test_3\\test_circuit_FMI\\sources\\ssc_core_9b671e57.c\" \"F:\\GitHubRepos\\FMI_test_3\\test_circuit_FMI\\sources\\ssc_core_9c016445.c\" \"F:\\GitHubRepos\\FMI_test_3\\test_circuit_FMI\\sources\\ssc_core_9c01d168.c\" \"F:\\GitHubRepos\\FMI_test_3\\test_circuit_FMI\\sources\\ssc_core_9dd110ad.c\" \"F:\\GitHubRepos\\FMI_test_3\\test_circuit_FMI\\sources\\ssc_core_9fb0e229.c\" \"F:\\GitHubRepos\\FMI_test_3\\test_circuit_FMI\\sources\\ssc_core_9fb25b4f.c\" \"F:\\GitHubRepos\\FMI_test_3\\test_circuit_FMI\\sources\\ssc_core_9fb2e56c.c\" \"F:\\GitHubRepos\\FMI_test_3\\test_circuit_FMI\\sources\\ssc_core_a1d393be.c\" \"F:\\GitHubRepos\\FMI_test_3\\test_circuit_FMI\\sources\\ssc_core_a269ab09.c\" \"F:\\GitHubRepos\\FMI_test_3\\test_circuit_FMI\\sources\\ssc_core_a4d4c45e.c\" \"F:\\GitHubRepos\\FMI_test_3\\test_circuit_FMI\\sources\\ssc_core_a4da1d0a.c\" \"F:\\GitHubRepos\\FMI_test_3\\test_circuit_FMI\\sources\\ssc_core_a6b78ccc.c\" \"F:\\GitHubRepos\\FMI_test_3\\test_circuit_FMI\\sources\\ssc_core_a76299bc.c\" \"F:\\GitHubRepos\\FMI_test_3\\test_circuit_FMI\\sources\\ssc_core_a867d880.c\" \"F:\\GitHubRepos\\FMI_test_3\\test_circuit_FMI\\sources\\ssc_core_a9bbaecc.c\" \"F:\\GitHubRepos\\FMI_test_3\\test_circuit_FMI\\sources\\ssc_core_a9bf1ff2.c\" \"F:\\GitHubRepos\\FMI_test_3\\test_circuit_FMI\\sources\\ssc_core_aa09f23c.c\" \"F:\\GitHubRepos\\FMI_test_3\\test_circuit_FMI\\sources\\ssc_core_abd05c18.c\" \"F:\\GitHubRepos\\FMI_test_3\\test_circuit_FMI\\sources\\ssc_core_abd5e7b4.c\" \"F:\\GitHubRepos\\FMI_test_3\\test_circuit_FMI\\sources\\ssc_core_acb64294.c\" \"F:\\GitHubRepos\\FMI_test_3\\test_circuit_FMI\\sources\\ssc_core_acb6462e.c\" \"F:\\GitHubRepos\\FMI_test_3\\test_circuit_FMI\\sources\\ssc_core_b1038cbb.c\" \"F:\\GitHubRepos\\FMI_test_3\\test_circuit_FMI\\sources\\ssc_core_b10e34f4.c\" \"F:\\GitHubRepos\\FMI_test_3\\test_circuit_FMI\\sources\\ssc_core_b2b3b239.c\" \"F:\\GitHubRepos\\FMI_test_3\\test_circuit_FMI\\sources\\ssc_core_b369cd13.c\" \"F:\\GitHubRepos\\FMI_test_3\\test_circuit_FMI\\sources\\ssc_core_b402b40d.c\" \"F:\\GitHubRepos\\FMI_test_3\\test_circuit_FMI\\sources\\ssc_core_b7b88213.c\" \"F:\\GitHubRepos\\FMI_test_3\\test_circuit_FMI\\sources\\ssc_core_b96ebc21.c\" \"F:\\GitHubRepos\\FMI_test_3\\test_circuit_FMI\\sources\\ssc_core_bad68669.c\" \"F:\\GitHubRepos\\FMI_test_3\\test_circuit_FMI\\sources\\ssc_core_bc648043.c\" \"F:\\GitHubRepos\\FMI_test_3\\test_circuit_FMI\\sources\\ssc_core_bfdb08db.c\" \"F:\\GitHubRepos\\FMI_test_3\\test_circuit_FMI\\sources\\ssc_core_c3003040.c\" \"F:\\GitHubRepos\\FMI_test_3\\test_circuit_FMI\\sources\\ssc_core_c5b050d7.c\" \"F:\\GitHubRepos\\FMI_test_3\\test_circuit_FMI\\sources\\ssc_core_c5b63cb2.c\" \"F:\\GitHubRepos\\FMI_test_3\\test_circuit_FMI\\sources\\ssc_core_c607b660.c\" \"F:\\GitHubRepos\\FMI_test_3\\test_circuit_FMI\\sources\\ssc_core_c8d83e88.c\" \"F:\\GitHubRepos\\FMI_test_3\\test_circuit_FMI\\sources\\ssc_core_cab615c8.c\" \"F:\\GitHubRepos\\FMI_test_3\\test_circuit_FMI\\sources\\ssc_core_cabdc251.c\" \"F:\\GitHubRepos\\FMI_test_3\\test_circuit_FMI\\sources\\ssc_core_cc067f58.c\" \"F:\\GitHubRepos\\FMI_test_3\\test_circuit_FMI\\sources\\ssc_core_cc0bcab0.c\" \"F:\\GitHubRepos\\FMI_test_3\\test_circuit_FMI\\sources\\ssc_core_ce6a84bb.c\" \"F:\\GitHubRepos\\FMI_test_3\\test_circuit_FMI\\sources\\ssc_core_d06d763c.c\" \"F:\\GitHubRepos\\FMI_test_3\\test_circuit_FMI\\sources\\ssc_core_d3d34d7c.c\" \"F:\\GitHubRepos\\FMI_test_3\\test_circuit_FMI\\sources\\ssc_core_d4b9397b.c\" \"F:\\GitHubRepos\\FMI_test_3\\test_circuit_FMI\\sources\\ssc_core_d70a6a09.c\" \"F:\\GitHubRepos\\FMI_test_3\\test_circuit_FMI\\sources\\ssc_core_d807fa59.c\" \"F:\\GitHubRepos\\FMI_test_3\\test_circuit_FMI\\sources\\ssc_core_dcda6edd.c\" \"F:\\GitHubRepos\\FMI_test_3\\test_circuit_FMI\\sources\\ssc_core_deb7fd8d.c\" \"F:\\GitHubRepos\\FMI_test_3\\test_circuit_FMI\\sources\\ssc_core_e0d0866d.c\" \"F:\\GitHubRepos\\FMI_test_3\\test_circuit_FMI\\sources\\ssc_core_e2b61d72.c\" \"F:\\GitHubRepos\\FMI_test_3\\test_circuit_FMI\\sources\\ssc_core_e400c1c2.c\" \"F:\\GitHubRepos\\FMI_test_3\\test_circuit_FMI\\sources\\ssc_core_ead8f455.c\" \"F:\\GitHubRepos\\FMI_test_3\\test_circuit_FMI\\sources\\ssc_core_edb836de.c\" \"F:\\GitHubRepos\\FMI_test_3\\test_circuit_FMI\\sources\\ssc_core_ee000fbe.c\" \"F:\\GitHubRepos\\FMI_test_3\\test_circuit_FMI\\sources\\ssc_core_ee01086d.c\" \"F:\\GitHubRepos\\FMI_test_3\\test_circuit_FMI\\sources\\ssc_core_ee0f0141.c\" \"F:\\GitHubRepos\\FMI_test_3\\test_circuit_FMI\\sources\\ssc_core_f9b6dbed.c\" \"F:\\GitHubRepos\\FMI_test_3\\test_circuit_FMI\\sources\\ssc_core_fa09e9e6.c\" \"F:\\GitHubRepos\\FMI_test_3\\test_circuit_FMI\\sources\\ssc_core_fbd34e62.c\" \"F:\\GitHubRepos\\FMI_test_3\\test_circuit_FMI\\sources\\ssc_core_ff06d9a4.c\" \"F:\\GitHubRepos\\FMI_test_3\\test_circuit_FMI\\sources\\ssc_st_7cd93bb6.c\" \"F:\\GitHubRepos\\FMI_test_3\\test_circuit_FMI\\sources\\ssc_st_da6cd8f8.c\" \"F:\\GitHubRepos\\FMI_test_3\\test_circuit_FMI\\sources\\mc_026e4f4b.c\" \"F:\\GitHubRepos\\FMI_test_3\\test_circuit_FMI\\sources\\mc_03b98f6f.c\" \"F:\\GitHubRepos\\FMI_test_3\\test_circuit_FMI\\sources\\mc_0764157d.c\" \"F:\\GitHubRepos\\FMI_test_3\\test_circuit_FMI\\sources\\mc_0bd30dee.c\" \"F:\\GitHubRepos\\FMI_test_3\\test_circuit_FMI\\sources\\mc_0d6fd085.c\" \"F:\\GitHubRepos\\FMI_test_3\\test_circuit_FMI\\sources\\mc_0ed73c49.c\" \"F:\\GitHubRepos\\FMI_test_3\\test_circuit_FMI\\sources\\mc_0edc34e3.c\" \"F:\\GitHubRepos\\FMI_test_3\\test_circuit_FMI\\sources\\mc_10d4ab75.c\" \"F:\\GitHubRepos\\FMI_test_3\\test_circuit_FMI\\sources\\mc_11086079.c\" \"F:\\GitHubRepos\\FMI_test_3\\test_circuit_FMI\\sources\\mc_110e6c6c.c\" \"F:\\GitHubRepos\\FMI_test_3\\test_circuit_FMI\\sources\\mc_1407e917.c\" \"F:\\GitHubRepos\\FMI_test_3\\test_circuit_FMI\\sources\\mc_140e3c4c.c\" \"F:\\GitHubRepos\\FMI_test_3\\test_circuit_FMI\\sources\\mc_15d12d95.c\" \"F:\\GitHubRepos\\FMI_test_3\\test_circuit_FMI\\sources\\mc_15d828ca.c\" \"F:\\GitHubRepos\\FMI_test_3\\test_circuit_FMI\\sources\\mc_220ba961.c\" \"F:\\GitHubRepos\\FMI_test_3\\test_circuit_FMI\\sources\\mc_2565d6e0.c\" \"F:\\GitHubRepos\\FMI_test_3\\test_circuit_FMI\\sources\\mc_2a642f54.c\" \"F:\\GitHubRepos\\FMI_test_3\\test_circuit_FMI\\sources\\mc_2a6a9b24.c\" \"F:\\GitHubRepos\\FMI_test_3\\test_circuit_FMI\\sources\\mc_2a6b417d.c\" \"F:\\GitHubRepos\\FMI_test_3\\test_circuit_FMI\\sources\\mc_2bbf87e3.c\" \"F:\\GitHubRepos\\FMI_test_3\\test_circuit_FMI\\sources\\mc_2cdc96b4.c\" \"F:\\GitHubRepos\\FMI_test_3\\test_circuit_FMI\\sources\\mc_32d501e3.c\" \"F:\\GitHubRepos\\FMI_test_3\\test_circuit_FMI\\sources\\mc_32dc008a.c\" \"F:\\GitHubRepos\\FMI_test_3\\test_circuit_FMI\\sources\\mc_3b6a945d.c\" \"F:\\GitHubRepos\\FMI_test_3\\test_circuit_FMI\\sources\\mc_3e66abdf.c\" \"F:\\GitHubRepos\\FMI_test_3\\test_circuit_FMI\\sources\\mc_4105189f.c\" \"F:\\GitHubRepos\\FMI_test_3\\test_circuit_FMI\\sources\\mc_47b8cebe.c\" \"F:\\GitHubRepos\\FMI_test_3\\test_circuit_FMI\\sources\\mc_47b91db1.c\" \"F:\\GitHubRepos\\FMI_test_3\\test_circuit_FMI\\sources\\mc_4b0301c6.c\" \"F:\\GitHubRepos\\FMI_test_3\\test_circuit_FMI\\sources\\mc_4c6117e3.c\" \"F:\\GitHubRepos\\FMI_test_3\\test_circuit_FMI\\sources\\mc_51d4094e.c\" \"F:\\GitHubRepos\\FMI_test_3\\test_circuit_FMI\\sources\\mc_52623861.c\" \"F:\\GitHubRepos\\FMI_test_3\\test_circuit_FMI\\sources\\mc_52688a58.c\" \"F:\\GitHubRepos\\FMI_test_3\\test_circuit_FMI\\sources\\mc_53b1fc84.c\" \"F:\\GitHubRepos\\FMI_test_3\\test_circuit_FMI\\sources\\mc_53b6fcf3.c\" \"F:\\GitHubRepos\\FMI_test_3\\test_circuit_FMI\\sources\\mc_550847c3.c\" \"F:\\GitHubRepos\\FMI_test_3\\test_circuit_FMI\\sources\\mc_5766048f.c\" \"F:\\GitHubRepos\\FMI_test_3\\test_circuit_FMI\\sources\\mc_59b6e413.c\" \"F:\\GitHubRepos\\FMI_test_3\\test_circuit_FMI\\sources\\mc_5bd2c9c1.c\" \"F:\\GitHubRepos\\FMI_test_3\\test_circuit_FMI\\sources\\mc_5d65cd86.c\" \"F:\\GitHubRepos\\FMI_test_3\\test_circuit_FMI\\sources\\mc_5edd42ef.c\" \"F:\\GitHubRepos\\FMI_test_3\\test_circuit_FMI\\sources\\mc_630208f8.c\" \"F:\\GitHubRepos\\FMI_test_3\\test_circuit_FMI\\sources\\mc_630dda0e.c\" \"F:\\GitHubRepos\\FMI_test_3\\test_circuit_FMI\\sources\\mc_67da200d.c\" \"F:\\GitHubRepos\\FMI_test_3\\test_circuit_FMI\\sources\\mc_67da4f41.c\" \"F:\\GitHubRepos\\FMI_test_3\\test_circuit_FMI\\sources\\mc_6b6d311a.c\" \"F:\\GitHubRepos\\FMI_test_3\\test_circuit_FMI\\sources\\mc_6e61d16c.c\" \"F:\\GitHubRepos\\FMI_test_3\\test_circuit_FMI\\sources\\mc_6fb1c336.c\" \"F:\\GitHubRepos\\FMI_test_3\\test_circuit_FMI\\sources\\mc_7207b6f4.c\" \"F:\\GitHubRepos\\FMI_test_3\\test_circuit_FMI\\sources\\mc_7809a65c.c\" \"F:\\GitHubRepos\\FMI_test_3\\test_circuit_FMI\\sources\\mc_7a613aec.c\" \"F:\\GitHubRepos\\FMI_test_3\\test_circuit_FMI\\sources\\mc_7bbf41f0.c\" \"F:\\GitHubRepos\\FMI_test_3\\test_circuit_FMI\\sources\\mc_7cd58f0b.c\" \"F:\\GitHubRepos\\FMI_test_3\\test_circuit_FMI\\sources\\mc_7cdbe436.c\" \"F:\\GitHubRepos\\FMI_test_3\\test_circuit_FMI\\sources\\mc_7d0547c8.c\" \"F:\\GitHubRepos\\FMI_test_3\\test_circuit_FMI\\sources\\mc_7d099de7.c\" \"F:\\GitHubRepos\\FMI_test_3\\test_circuit_FMI\\sources\\mc_7eb21b39.c\" \"F:\\GitHubRepos\\FMI_test_3\\test_circuit_FMI\\sources\\mc_81b0ada5.c\" \"F:\\GitHubRepos\\FMI_test_3\\test_circuit_FMI\\sources\\mc_81b5717e.c\" \"F:\\GitHubRepos\\FMI_test_3\\test_circuit_FMI\\sources\\mc_81bc7943.c\" \"F:\\GitHubRepos\\FMI_test_3\\test_circuit_FMI\\sources\\mc_870ec75e.c\" \"F:\\GitHubRepos\\FMI_test_3\\test_circuit_FMI\\sources\\mc_89d597cf.c\" \"F:\\GitHubRepos\\FMI_test_3\\test_circuit_FMI\\sources\\mc_90b6aa0a.c\" \"F:\\GitHubRepos\\FMI_test_3\\test_circuit_FMI\\sources\\mc_95b62b73.c\" \"F:\\GitHubRepos\\FMI_test_3\\test_circuit_FMI\\sources\\mc_9ab7d9b0.c\" \"F:\\GitHubRepos\\FMI_test_3\\test_circuit_FMI\\sources\\mc_9b6376d1.c\" \"F:\\GitHubRepos\\FMI_test_3\\test_circuit_FMI\\sources\\mc_9b6c1529.c\" \"F:\\GitHubRepos\\FMI_test_3\\test_circuit_FMI\\sources\\mc_a2647600.c\" \"F:\\GitHubRepos\\FMI_test_3\\test_circuit_FMI\\sources\\mc_a26bab1a.c\" \"F:\\GitHubRepos\\FMI_test_3\\test_circuit_FMI\\sources\\mc_a3b90582.c\" \"F:\\GitHubRepos\\FMI_test_3\\test_circuit_FMI\\sources\\mc_a6b5ed24.c\" \"F:\\GitHubRepos\\FMI_test_3\\test_circuit_FMI\\sources\\mc_a7684938.c\" \"F:\\GitHubRepos\\FMI_test_3\\test_circuit_FMI\\sources\\mc_a865d1dd.c\" \"F:\\GitHubRepos\\FMI_test_3\\test_circuit_FMI\\sources\\mc_acb3fad7.c\" \"F:\\GitHubRepos\\FMI_test_3\\test_circuit_FMI\\sources\\mc_af0bc203.c\" \"F:\\GitHubRepos\\FMI_test_3\\test_circuit_FMI\\sources\\mc_af0cc4c9.c\" \"F:\\GitHubRepos\\FMI_test_3\\test_circuit_FMI\\sources\\mc_b0de9cbc.c\" \"F:\\GitHubRepos\\FMI_test_3\\test_circuit_FMI\\sources\\mc_b2b86ae3.c\" \"F:\\GitHubRepos\\FMI_test_3\\test_circuit_FMI\\sources\\mc_b362c5eb.c\" \"F:\\GitHubRepos\\FMI_test_3\\test_circuit_FMI\\sources\\mc_b7b03d44.c\" \"F:\\GitHubRepos\\FMI_test_3\\test_circuit_FMI\\sources\\mc_b96a0bad.c\" \"F:\\GitHubRepos\\FMI_test_3\\test_circuit_FMI\\sources\\mc_bb0520ee.c\" \"F:\\GitHubRepos\\FMI_test_3\\test_circuit_FMI\\sources\\mc_bdbb9b78.c\" \"F:\\GitHubRepos\\FMI_test_3\\test_circuit_FMI\\sources\\mc_c2dbf4b2.c\" \"F:\\GitHubRepos\\FMI_test_3\\test_circuit_FMI\\sources\\mc_c8d25d23.c\" \"F:\\GitHubRepos\\FMI_test_3\\test_circuit_FMI\\sources\\mc_cab8a1f9.c\" \"F:\\GitHubRepos\\FMI_test_3\\test_circuit_FMI\\sources\\mc_ce6656ce.c\" \"F:\\GitHubRepos\\FMI_test_3\\test_circuit_FMI\\sources\\mc_d20085b7.c\" \"F:\\GitHubRepos\\FMI_test_3\\test_circuit_FMI\\sources\\mc_d9d38185.c\" \"F:\\GitHubRepos\\FMI_test_3\\test_circuit_FMI\\sources\\mc_dbbb14d2.c\" \"F:\\GitHubRepos\\FMI_test_3\\test_circuit_FMI\\sources\\mc_dcdddfae.c\" \"F:\\GitHubRepos\\FMI_test_3\\test_circuit_FMI\\sources\\mc_debb448f.c\" \"F:\\GitHubRepos\\FMI_test_3\\test_circuit_FMI\\sources\\mc_e7b99cf6.c\" \"F:\\GitHubRepos\\FMI_test_3\\test_circuit_FMI\\sources\\mc_e7bc2f1a.c\" \"F:\\GitHubRepos\\FMI_test_3\\test_circuit_FMI\\sources\\mc_e9661c4a.c\" \"F:\\GitHubRepos\\FMI_test_3\\test_circuit_FMI\\sources\\mc_e969ae87.c\" \"F:\\GitHubRepos\\FMI_test_3\\test_circuit_FMI\\sources\\mc_edbf543c.c\" \"F:\\GitHubRepos\\FMI_test_3\\test_circuit_FMI\\sources\\mc_ee000fbe.c\" \"F:\\GitHubRepos\\FMI_test_3\\test_circuit_FMI\\sources\\mc_efdea3a7.c\" \"F:\\GitHubRepos\\FMI_test_3\\test_circuit_FMI\\sources\\mc_f0012953.c\" \"F:\\GitHubRepos\\FMI_test_3\\test_circuit_FMI\\sources\\mc_f00d2f9b.c\" \"F:\\GitHubRepos\\FMI_test_3\\test_circuit_FMI\\sources\\mc_f3be157c.c\" \"F:\\GitHubRepos\\FMI_test_3\\test_circuit_FMI\\sources\\mc_fbd54145.c\" \"F:\\GitHubRepos\\FMI_test_3\\test_circuit_FMI\\sources\\mc_fcb15a9b.c\" \"F:\\GitHubRepos\\FMI_test_3\\test_circuit_FMI\\sources\\mc_fd619d14.c\" \"F:\\GitHubRepos\\FMI_test_3\\test_circuit_FMI\\sources\\mc_fd6341bb.c\" \"F:\\GitHubRepos\\FMI_test_3\\test_circuit_FMI\\sources\\ex_04d5441d.c\" \"F:\\GitHubRepos\\FMI_test_3\\test_circuit_FMI\\sources\\ex_0d6d0784.c\" \"F:\\GitHubRepos\\FMI_test_3\\test_circuit_FMI\\sources\\ex_136645f8.c\" \"F:\\GitHubRepos\\FMI_test_3\\test_circuit_FMI\\sources\\ex_17bc61ac.c\" \"F:\\GitHubRepos\\FMI_test_3\\test_circuit_FMI\\sources\\ex_18b4440a.c\" \"F:\\GitHubRepos\\FMI_test_3\\test_circuit_FMI\\sources\\ex_1b03ca17.c\" \"F:\\GitHubRepos\\FMI_test_3\\test_circuit_FMI\\sources\\ex_2ebcd5b2.c\" \"F:\\GitHubRepos\\FMI_test_3\\test_circuit_FMI\\sources\\ex_316a81de.c\" \"F:\\GitHubRepos\\FMI_test_3\\test_circuit_FMI\\sources\\ex_36012fa7.c\" \"F:\\GitHubRepos\\FMI_test_3\\test_circuit_FMI\\sources\\ex_40d5be33.c\" \"F:\\GitHubRepos\\FMI_test_3\\test_circuit_FMI\\sources\\ex_47b11894.c\" \"F:\\GitHubRepos\\FMI_test_3\\test_circuit_FMI\\sources\\ex_57660158.c\" \"F:\\GitHubRepos\\FMI_test_3\\test_circuit_FMI\\sources\\ex_690b7cd0.c\" \"F:\\GitHubRepos\\FMI_test_3\\test_circuit_FMI\\sources\\ex_6dd8e72d.c\" \"F:\\GitHubRepos\\FMI_test_3\\test_circuit_FMI\\sources\\ex_770385e6.c\" \"F:\\GitHubRepos\\FMI_test_3\\test_circuit_FMI\\sources\\ex_79d100f1.c\" \"F:\\GitHubRepos\\FMI_test_3\\test_circuit_FMI\\sources\\ex_8a6fc761.c\" \"F:\\GitHubRepos\\FMI_test_3\\test_circuit_FMI\\sources\\ex_98d223a6.c\" \"F:\\GitHubRepos\\FMI_test_3\\test_circuit_FMI\\sources\\ex_aed5de1e.c\" \"F:\\GitHubRepos\\FMI_test_3\\test_circuit_FMI\\sources\\ex_b2b40ad5.c\" \"F:\\GitHubRepos\\FMI_test_3\\test_circuit_FMI\\sources\\ex_bb0efd4b.c\" \"F:\\GitHubRepos\\FMI_test_3\\test_circuit_FMI\\sources\\ex_bfdb009c.c\" \"F:\\GitHubRepos\\FMI_test_3\\test_circuit_FMI\\sources\\ex_c9069dae.c\" \"F:\\GitHubRepos\\FMI_test_3\\test_circuit_FMI\\sources\\ex_d9d686a8.c\" \"F:\\GitHubRepos\\FMI_test_3\\test_circuit_FMI\\sources\\ex_debffef2.c\" \"F:\\GitHubRepos\\FMI_test_3\\test_circuit_FMI\\sources\\ex_e40d74b8.c\" \"F:\\GitHubRepos\\FMI_test_3\\test_circuit_FMI\\sources\\ex_eb0d559b.c\" \"F:\\GitHubRepos\\FMI_test_3\\test_circuit_FMI\\sources\\ex_f6bb4c2d.c\" \"F:\\GitHubRepos\\FMI_test_3\\test_circuit_FMI\\sources\\ex_f866102d.c\" \"F:\\GitHubRepos\\FMI_test_3\\test_circuit_FMI\\sources\\slu_stubbed_definitions.c\" \"F:\\GitHubRepos\\FMI_test_3\\test_circuit_FMI\\sources\\pm_09bc42e2.c\" \"F:\\GitHubRepos\\FMI_test_3\\test_circuit_FMI\\sources\\pm_14098e54.c\" \"F:\\GitHubRepos\\FMI_test_3\\test_circuit_FMI\\sources\\pm_26dc3230.c\" \"F:\\GitHubRepos\\FMI_test_3\\test_circuit_FMI\\sources\\pm_4fd5f5b9.c\" \"F:\\GitHubRepos\\FMI_test_3\\test_circuit_FMI\\sources\\pm_fed8c2c9.c\""  GenerateWebview=on  GenerateCodeMetricsReport=on
settings CodeAppCC: ForceParamTrailComments=on  IgnoreCustomStorageClasses=off  OperatorAnnotations=on  SimulinkDataObjDesc=on  SFDataObjDesc=on  MATLABFcnDesc=on  InsertBlockDesc=on  StateflowObjectComments=on  MATLABSourceComments=on  ReqsInCode=on
settings ERTTargetCC: TargetLangStandard=C99 (ISO)  GenerateSampleERTMain=on  CodeInterfacePackaging=Reusable function  SupportContinuousTime=on  InlinedParameterPlacement=NonHierarchical  RTWCAPISignals=on  RTWCAPIParams=on  RTWCAPIStates=on  RTWCAPIRootIO=on  ERTCustomFileTemplate=example_file_process.tlc

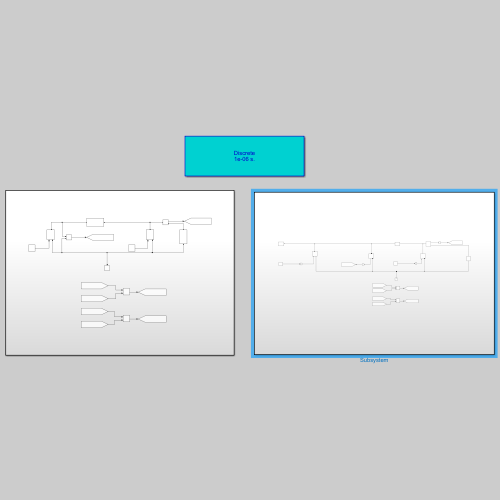
[thumbnail: Simulink's stored preview of the top-level diagram]
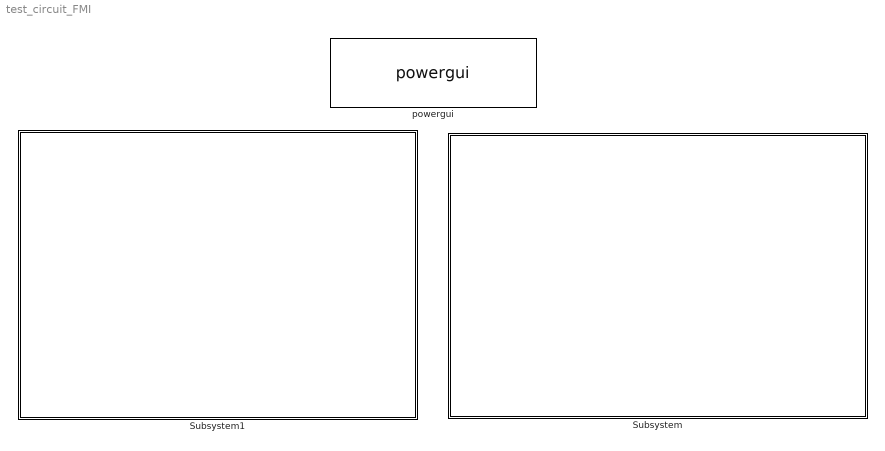
== system test_circuit_FMI ==
  Subsystem : Subsystem
  Subsystem1 : Subsystem
  powergui : spspowerguiLib/powergui  Priority=1  SimulationMode=Discrete  SampleTime=1e-6  frequency=60  Iterations=50  frequencyindice=0  Pbase=100e6  ErrMax=1e-4  UnitsV=kV  UnitsW=MW  buscounter=0  FunctionMessages=off  echomessages=off  EnableUseOfTLC=off  CurrentSourceSwitches=off  DisableSnubberDevices=off  DisableRonSwitches=off  DisableVfSwitches=off  DisplayEquations=off  AutomaticDiscreteSolvers=off  SolverType=Tustin/Backward Euler (TBE)  Interpol=off  ExternalGateDelay=off  methode=off  Ts=100  x0status=blocks  SPID=on  SwTol=0  HookPort=off  NonlinearTolerance=1e-4  nMaxIteration=100  ContinueOnMaxIteration=off  RestoreLinks=warning  ResistiveCurrentMeasurement=off  Frange=[0:2:500]  Ylog=off  Xlog=on  ShowGrid=off  save=off  variable=ZData  structure=0  ZoomFFT=off  StartTime=0.0  cycles=1  DisplayStyle=1  fundamental=60  FreqAxis=off  MaxFrequency=1000  frequencyindicesteady=1  RmsSteady=1  display=off
